simulink model "algebraic_design_model"  (R2023b)
settings: Solver=VariableStepAuto  StartTime=0.0  StopTime=4  MaxStep=0.001 * Ts  MinStep=0.0001 * Ts  RelTol=1e-3
values from neighbouring files (symbols this model uses):
  Ts = 50e-3    (= 0.05)    [MPC_design.m]    (also in algebraic_design.m = 0.002; quiz1.m = 1; quiz2.m = 1; quiz3.m = 0.002)
libraries: cstblocks x3, simulink x1
settings Model: Creator=lucap  LastModifiedBy=lucap

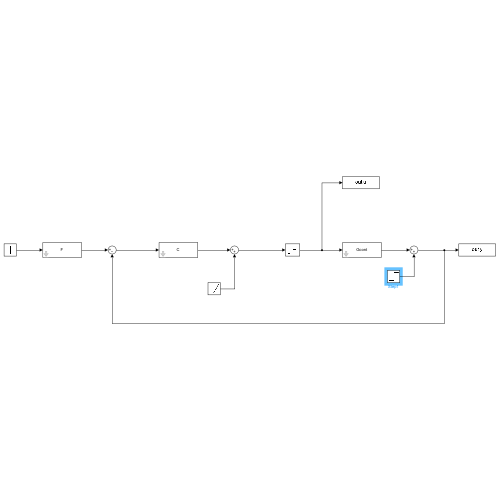
[thumbnail: Simulink's stored preview of the top-level diagram]
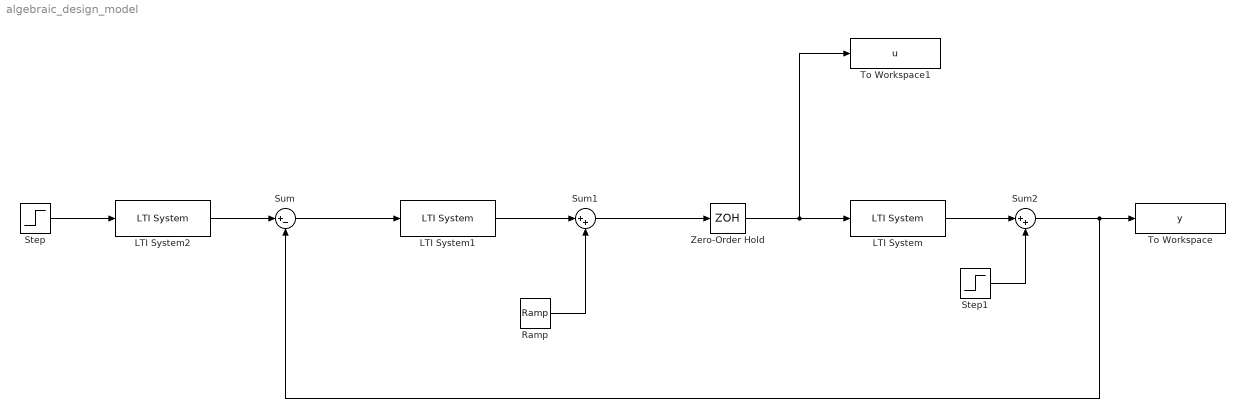
== system algebraic_design_model ==
  LTI System : cstblocks/LTI System  sys=Gcont  IC=[]  PadeOrder=0
  LTI System1 : cstblocks/LTI System  sys=C  IC=[]  PadeOrder=0
  LTI System2 : cstblocks/LTI System  sys=F  IC=[]  PadeOrder=0
  Ramp : simulink/Sources/Ramp  slope=0  start=0  InitialOutput=0
  Step : Step  Time=0  After=0  SampleTime=0
  Step1 : Step  Time=0  After=2  SampleTime=0
  Sum : Sum  Inputs=|+-
  Sum1 : Sum  Inputs=|++
  Sum2 : Sum  Inputs=|++
  To Workspace : ToWorkspace  VariableName=y  SaveFormat=Timeseries  SampleTime=Ts * 0.001
  To Workspace1 : ToWorkspace  VariableName=u  SaveFormat=Timeseries  SampleTime=Ts * 0.001
  Zero-Order Hold : ZeroOrderHold  SampleTime=Ts
  wires:
  Sum/1 -> LTI System1/1
  LTI System1/1 -> Sum1/1
  LTI System/1 -> Sum2/1
  Sum2/1 -> Sum/2, To Workspace/1
  Step1/1 -> Sum2/2
  Step/1 -> LTI System2/1
  LTI System2/1 -> Sum/1
  Ramp/1 -> Sum1/2
  Sum1/1 -> Zero-Order Hold/1
  Zero-Order Hold/1 -> To Workspace1/1, LTI System/1
